simulink model "model"  (R2022b)
settings: Solver=VariableStepAuto  StartTime=0.0  StopTime=10  RelTol=1e-3
libraries: fuzblock x4, slpidlib x2
settings Model: Creator=Lenovo  LastModifiedBy=Lenovo

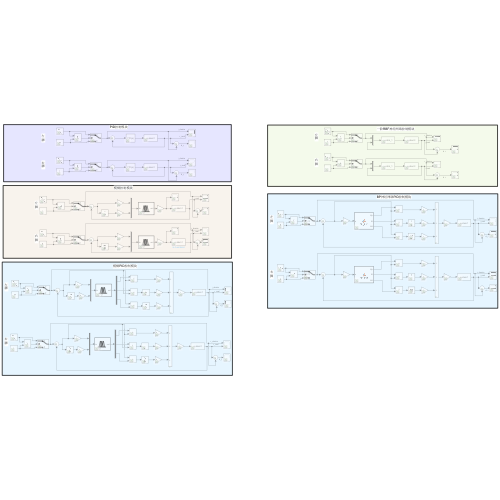
[thumbnail: Simulink's stored preview of the top-level diagram]
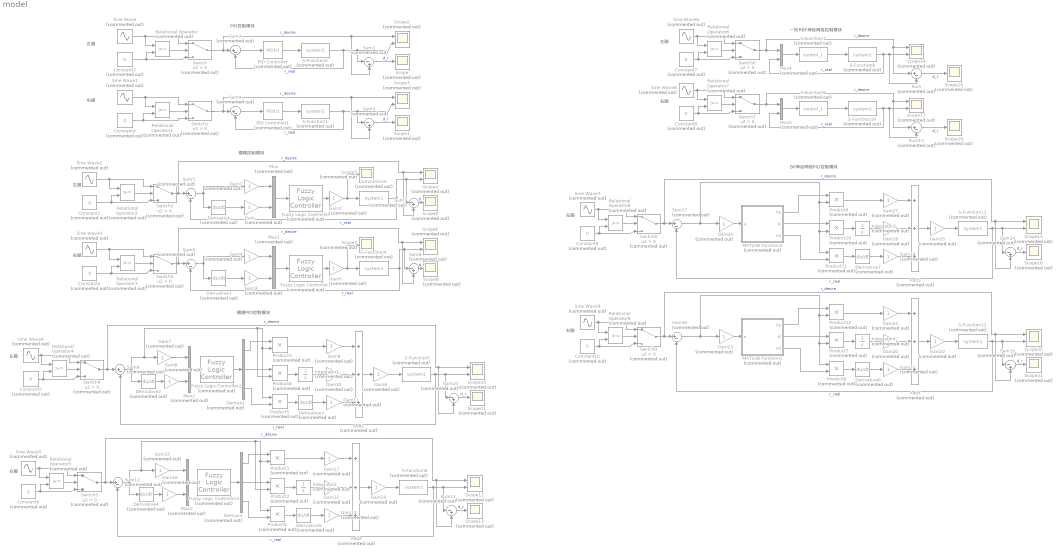
== system model ==
  note: 左脚
  note: PID控制模块
  note: 右脚
  note: 模糊控制模块
  note: 左脚
  note: 右脚
  note: 模糊PID控制模块
  note: 左脚
  note: 右脚
  note: 一阶RBF神经网络控制模块
  note: 左脚
  note: 右脚
  note: BP神经网络PID控制模块
  note: 左脚
  note: 右脚
  Add{1..4} (4 alike) : Sum  Commented=on  Inputs=+++
  Constant{1..10} (10 alike) : Constant  Commented=on  Value=0
  Demux1 : Demux  Commented=on  Outputs=3
  Demux2 : Demux  Commented=on  Outputs=3
  Derivative{,1..7} (8 alike) : Derivative  Commented=on
  Fuzzy Logic Controller : fuzblock/Fuzzy Logic  Controller  Commented=on  FIS='fuzzy1.fis'  OutputSampleNumber=101  DataType=double  FuzzifiedInputs=off  RuleFiringStrengths=off  RuleOutputs=off  AggregatedOutputs=off  SimulateUsing=Interpreted execution  OutOfRangeInputValueMessage=warning  NoRuleFiredMessage=warning  EmptyOutputFuzzySetMessage=warning
  Fuzzy Logic Controller1 : fuzblock/Fuzzy Logic  Controller  Commented=on  FIS='fuzzy1.fis'  OutputSampleNumber=101  DataType=double  FuzzifiedInputs=off  RuleFiringStrengths=off  RuleOutputs=off  AggregatedOutputs=off  SimulateUsing=Interpreted execution  OutOfRangeInputValueMessage=warning  NoRuleFiredMessage=warning  EmptyOutputFuzzySetMessage=warning
  Fuzzy Logic Controller2 : fuzblock/Fuzzy Logic  Controller  Commented=on  FIS='PIDfuzzy1.fis'  OutputSampleNumber=101  DataType=double  FuzzifiedInputs=off  RuleFiringStrengths=off  RuleOutputs=off  AggregatedOutputs=off  SimulateUsing=Interpreted execution  OutOfRangeInputValueMessage=warning  NoRuleFiredMessage=warning  EmptyOutputFuzzySetMessage=warning
  Fuzzy Logic Controller3 : fuzblock/Fuzzy Logic  Controller  Commented=on  FIS='PIDfuzzy1.fis'  OutputSampleNumber=101  DataType=double  FuzzifiedInputs=off  RuleFiringStrengths=off  RuleOutputs=off  AggregatedOutputs=off  SimulateUsing=Interpreted execution  OutOfRangeInputValueMessage=warning  NoRuleFiredMessage=warning  EmptyOutputFuzzySetMessage=warning
  Gain{,1..27} (28 alike) : Gain  Commented=on
  Integrator{1..4} (4 alike) : Integrator  Commented=on
  MATLAB Function1 : MATLAB Function  Commented=on  TreatAsAtomicUnit=on
  MATLAB Function2 : MATLAB Function  Commented=on  TreatAsAtomicUnit=on
  Mux{,1..5} (6 alike) : Mux  Commented=on  Inputs=2
  PID Controller : slpidlib/PID Controller  Commented=on  Controller=PID  Form=Parallel  TimeDomain=Continuous-time  UseExternalTs=off  SampleTime=-1  IntegratorMethod=Forward Euler  FilterMethod=Forward Euler  ControllerParametersSource=internal  P=871.012527892708  I=1996.38268425314  UseKiTs=off  D=84.4356751014045  N=44899.2539327158  UseFilter=on  TunerSelectOption=Transfer Function Based (PID Tuner App)  InitialConditionSource=internal  InitialConditionForIntegrator=0  InitialConditionForFilter=0  DifferentiatorICPrevScaledInput=0  ExternalReset=none  TrackingMode=off  Kt=1  LimitOutput=off  SatLimitsSource=internal  UpperSaturationLimit=inf  LowerSaturationLimit=-inf  LinearizeAsGain=on  AntiWindupMode=none  Kb=1  LimitIntegrator=off  UpperIntegratorSaturationLimit=inf  LowerIntegratorSaturationLimit=-inf  POutMin=[]  POutMax=[]  IOutMin=[]  IOutMax=[]  DOutMin=[]  DOutMax=[]  NOutMin=[]  NOutMax=[]  SumOutMin=[]  SumOutMax=[]  SaturationOutMin=[]  SaturationOutMax=[]  PParamMin=[]  PParamMax=[]  IParamMin=[]  IParamMax=[]  DParamMin=[]  DParamMax=[]  NParamMin=[]  NParamMax=[]  KbParamMin=[]  KbParamMax=[]  KtParamMin=[]  KtParamMax=[]  KbOutMin=[]  KbOutMax=[]  KtOutMin=[]  KtOutMax=[]  IntegratorOutMin=[]  IntegratorOutMax=[]  FilterOutMin=[]  FilterOutMax=[]  SumI1OutMin=[]  SumI1OutMax=[]  SumI2OutMin=[]  SumI2OutMax=[]  SumI3OutMin=[]  SumI3OutMax=[]  SumI4OutMin=[]  SumI4OutMax=[]  SumDOutMin=[]  SumDOutMax=[]  DifferentiatorOutMin=[]  DifferentiatorOutMax=[]  FilterDiffOutCoefMin=[]  FilterDiffOutCoefMax=[]  ReciprocalOutMin=[]  ReciprocalOutMax=[]  SumDenOutMin=[]  SumDenOutMax=[]  SumNumOutMin=[]  SumNumOutMax=[]  DivideOutMin=[]  DivideOutMax=[]  UdiffTsProdOutMin=[]  UdiffTsProdOutMax=[]  NTsProdOutMin=[]  NTsProdOutMax=[]  UintegralTsProdOutMin=[]  UintegralTsProdOutMax=[]  UngainTsProdOutMin=[]  UngainTsProdOutMax=[]  ClampingZeroOutDataTypeStr=Inherit: Inherit via back propagation  ClampingZeroOutMin=[]  ClampingZeroOutMax=[]  FilterDenConstantOutDataTypeStr=Inherit: Inherit via back propagation  FilterDenConstantOutMin=[]  FilterDenConstantOutMax=[]  PCopyOutDataTypeStr=Inherit: Inherit via back propagation  PCopyOutMin=[]  PCopyOutMax=[]  NCopyOutDataTypeStr=Inherit: Inherit via back propagation  NCopyOutMin=[]  NCopyOutMax=[]  IntegratorContinuousStateAttributes=''  IntegratorStateMustResolveToSignalObject=off  IntegratorRTWStateStorageClass=Auto  FilterContinuousStateAttributes=''  FilterStateMustResolveToSignalObject=off  FilterRTWStateStorageClass=Auto  ParallelPVariant=InternalParameters  IdealPVariant=Disabled  IVariant=InternalParameters  DVariant=InternalParameters  IntegratorVariant=Continuous  SatVariant=Disabled  AWVariant=Passthrough  PCopyVariant=Disabled  TRVariant=Disabled  FdbkBlocksVariant=Forward  IdealPFdbkVariant=Disabled  SatFdbkVariant=Disabled  DerivativeFilterVariant=ContFilter  NVariant=InternalParameters  NCopyVariant=Disabled  FilterICVariant=InternalICsFilter  IntegratorICVariant=InternalICs  ExternalResetVariant=Disabled  TRSumVariant=Passthrough  SumFdbkVariant=Disabled  SumVariant=Sum_PID  TsampFilterVariant=InternalTs  TsampNgainVariant=Passthrough  TsampIntegralVariant=Passthrough  ExternalSaturationOutDataTypeStr=Inherit: Same as second input
  PID Controller1 : slpidlib/PID Controller  Commented=on  Controller=PID  Form=Parallel  TimeDomain=Continuous-time  UseExternalTs=off  SampleTime=-1  IntegratorMethod=Forward Euler  FilterMethod=Forward Euler  ControllerParametersSource=internal  P=871.012527892708  I=1996.38268425314  UseKiTs=off  D=84.4356751014045  N=44899.2539327158  UseFilter=on  TunerSelectOption=Transfer Function Based (PID Tuner App)  InitialConditionSource=internal  InitialConditionForIntegrator=0  InitialConditionForFilter=0  DifferentiatorICPrevScaledInput=0  ExternalReset=none  TrackingMode=off  Kt=1  LimitOutput=off  SatLimitsSource=internal  UpperSaturationLimit=inf  LowerSaturationLimit=-inf  LinearizeAsGain=on  AntiWindupMode=none  Kb=1  LimitIntegrator=off  UpperIntegratorSaturationLimit=inf  LowerIntegratorSaturationLimit=-inf  POutMin=[]  POutMax=[]  IOutMin=[]  IOutMax=[]  DOutMin=[]  DOutMax=[]  NOutMin=[]  NOutMax=[]  SumOutMin=[]  SumOutMax=[]  SaturationOutMin=[]  SaturationOutMax=[]  PParamMin=[]  PParamMax=[]  IParamMin=[]  IParamMax=[]  DParamMin=[]  DParamMax=[]  NParamMin=[]  NParamMax=[]  KbParamMin=[]  KbParamMax=[]  KtParamMin=[]  KtParamMax=[]  KbOutMin=[]  KbOutMax=[]  KtOutMin=[]  KtOutMax=[]  IntegratorOutMin=[]  IntegratorOutMax=[]  FilterOutMin=[]  FilterOutMax=[]  SumI1OutMin=[]  SumI1OutMax=[]  SumI2OutMin=[]  SumI2OutMax=[]  SumI3OutMin=[]  SumI3OutMax=[]  SumI4OutMin=[]  SumI4OutMax=[]  SumDOutMin=[]  SumDOutMax=[]  DifferentiatorOutMin=[]  DifferentiatorOutMax=[]  FilterDiffOutCoefMin=[]  FilterDiffOutCoefMax=[]  ReciprocalOutMin=[]  ReciprocalOutMax=[]  SumDenOutMin=[]  SumDenOutMax=[]  SumNumOutMin=[]  SumNumOutMax=[]  DivideOutMin=[]  DivideOutMax=[]  UdiffTsProdOutMin=[]  UdiffTsProdOutMax=[]  NTsProdOutMin=[]  NTsProdOutMax=[]  UintegralTsProdOutMin=[]  UintegralTsProdOutMax=[]  UngainTsProdOutMin=[]  UngainTsProdOutMax=[]  ClampingZeroOutDataTypeStr=Inherit: Inherit via back propagation  ClampingZeroOutMin=[]  ClampingZeroOutMax=[]  FilterDenConstantOutDataTypeStr=Inherit: Inherit via back propagation  FilterDenConstantOutMin=[]  FilterDenConstantOutMax=[]  PCopyOutDataTypeStr=Inherit: Inherit via back propagation  PCopyOutMin=[]  PCopyOutMax=[]  NCopyOutDataTypeStr=Inherit: Inherit via back propagation  NCopyOutMin=[]  NCopyOutMax=[]  IntegratorContinuousStateAttributes=''  IntegratorStateMustResolveToSignalObject=off  IntegratorRTWStateStorageClass=Auto  FilterContinuousStateAttributes=''  FilterStateMustResolveToSignalObject=off  FilterRTWStateStorageClass=Auto  ParallelPVariant=InternalParameters  IdealPVariant=Disabled  IVariant=InternalParameters  DVariant=InternalParameters  IntegratorVariant=Continuous  SatVariant=Disabled  AWVariant=Passthrough  PCopyVariant=Disabled  TRVariant=Disabled  FdbkBlocksVariant=Forward  IdealPFdbkVariant=Disabled  SatFdbkVariant=Disabled  DerivativeFilterVariant=ContFilter  NVariant=InternalParameters  NCopyVariant=Disabled  FilterICVariant=InternalICsFilter  IntegratorICVariant=InternalICs  ExternalResetVariant=Disabled  TRSumVariant=Passthrough  SumFdbkVariant=Disabled  SumVariant=Sum_PID  TsampFilterVariant=InternalTs  TsampNgainVariant=Passthrough  TsampIntegralVariant=Passthrough  ExternalSaturationOutDataTypeStr=Inherit: Same as second input
  Product{1..12} (12 alike) : Product  Commented=on
  Relational Operator{,1..9} (10 alike) : RelationalOperator  Commented=on  OutDataTypeStr=boolean  RndMeth=Simplest  InputSameDT=off
  S-Function{1..6,8,10..12} (10 alike) : S-Function  Commented=on  FunctionName=system1  SFunctionDeploymentMode=off  EnableBusSupport=off
  S-Function7 : S-Function  Commented=on  FunctionName=control_1  SFunctionDeploymentMode=off  EnableBusSupport=off
  S-Function9 : S-Function  Commented=on  FunctionName=control_1  SFunctionDeploymentMode=off  EnableBusSupport=off
  Scope{,1,5,7..9,11,13,16,18..19,21} (12 alike) : Scope  Commented=on
  Scope{2..4,6,10,12,14..15,17,20} (10 alike) : Scope  Commented=on  NumInputPorts=2
  Sine Wave{,2,4,6..7} (5 alike) : Sin  Commented=on  SampleTime=0
  Sine Wave{1,3,5,8..9} (5 alike) : Sin  Commented=on  Phase=pi  SampleTime=0
  Sum{,2,4..6,9,12..13,16..17} (10 alike) : Sum  Commented=on  Inputs=|+-
  Sum{1,3,7..8,10..11,14..15} (8 alike) : Sum  Commented=on  Inputs=|-+
  Switch{,1..9} (10 alike) : Switch  Commented=on  Criteria=u2 > Threshold  SaturateOnIntegerOverflow=off  InputSameDT=off
  wires:
  S-Function2/1 -> Scope2/2, Sum1/1, Sum2/2  "r_real"
  Switch/1 -> Scope2/1, Sum1/2, Sum2/1  "r_desire"
  PID Controller/1 -> S-Function2/1
  Sum2/1 -> PID Controller/1
  Sum1/1 -> Scope/1  "d_r"
  Switch1/1 -> Scope3/1, Sum3/2, Sum4/1  "r_desire"
  PID Controller1/1 -> S-Function1/1
  Sum3/1 -> Scope1/1  "d_r"
  S-Function1/1 -> Sum3/1, Scope3/2, Sum4/2  "r_real"
  Sum4/1 -> PID Controller1/1
  Relational Operator/1 -> Switch/2
  Sine Wave/1 -> Switch/1, Relational Operator/1
  Constant3/1 -> Relational Operator/2, Switch/3
  Relational Operator1/1 -> Switch1/2
  Sine Wave1/1 -> Switch1/1, Relational Operator1/1
  Constant4/1 -> Switch1/3, Relational Operator1/2
  Gain2/1 -> Scope5/1, S-Function3/1
  Derivative/1 -> Gain/1
  Gain/1 -> Mux/2
  Gain1/1 -> Mux/1
  S-Function3/1 -> Scope4/2, Sum7/1, Sum5/2  "r_real"
  Mux/1 -> Fuzzy Logic Controller/1
  Switch2/1 -> Sum7/2, Scope4/1, Sum5/1  "r_desire"
  Sum5/1 -> Derivative/1, Gain1/1
  Fuzzy Logic Controller/1 -> Gain2/1
  Sine Wave2/1 -> Switch2/1, Relational Operator2/1
  Relational Operator2/1 -> Switch2/2
  Constant1/1 -> Relational Operator2/2, Switch2/3
  Switch3/1 -> Scope6/1, Sum8/2, Sum6/1  "r_desire"
  Constant2/1 -> Relational Operator3/2, Switch3/3
  Relational Operator3/1 -> Switch3/2
  Sum6/1 -> Derivative1/1, Gain4/1
  Fuzzy Logic Controller1/1 -> Gain5/1
  Mux1/1 -> Fuzzy Logic Controller1/1
  Gain5/1 -> Scope7/1, S-Function4/1
  Gain3/1 -> Mux1/2
  Sine Wave3/1 -> Switch3/1, Relational Operator3/1
  Gain4/1 -> Mux1/1
  S-Function4/1 -> Sum6/2, Sum8/1, Scope6/2  "r_real"
  Derivative1/1 -> Gain3/1
  Sum7/1 -> Scope9/1  "d_r"
  Sum8/1 -> Scope8/1  "d_r"
  Derivative3/1 -> Gain11/1
  Gain8/1 -> Mux2/2
  Product4/1 -> Integrator1/1
  Product3/1 -> Gain9/1
  Add1/1 -> Gain6/1
  Sum9/1 -> Derivative2/1, Product5/1, Product3/2, Product4/2, Gain7/1
  Demux2/2 -> Product4/1
  Demux2/3 -> Product5/2
  Derivative2/1 -> Gain8/1
  Demux2/1 -> Product3/1
  Integrator1/1 -> Gain10/1
  Product5/1 -> Derivative3/1
  Gain7/1 -> Mux2/1
  Gain6/1 -> S-Function5/1
  Fuzzy Logic Controller2/1 -> Demux2/1
  S-Function5/1 -> Sum9/2, Sum10/1, Scope10/2  "r_real"
  Gain11/1 -> Add1/3
  Mux2/1 -> Fuzzy Logic Controller2/1
  Gain10/1 -> Add1/2
  Gain9/1 -> Add1/1
  Sine Wave4/1 -> Switch4/1, Relational Operator4/1
  Relational Operator4/1 -> Switch4/2
  Constant5/1 -> Relational Operator4/2, Switch4/3
  Sum10/1 -> Scope11/1  "d_r"
  Switch4/1 -> Sum10/2, Scope10/1, Sum9/1  "r_desire"
  Constant6/1 -> Relational Operator5/2, Switch5/3
  Sine Wave5/1 -> Switch5/1, Relational Operator5/1
  Relational Operator5/1 -> Switch5/2
  Sum11/1 -> Scope13/1  "d_r"
  Gain14/1 -> S-Function6/1
  Switch5/1 -> Sum11/2, Scope12/1, Sum12/1  "r_desire"
  Mux3/1 -> Fuzzy Logic Controller3/1
  Gain13/1 -> Add2/3
  Fuzzy Logic Controller3/1 -> Demux1/1
  S-Function6/1 -> Sum12/2, Sum11/1, Scope12/2  "r_real"
  Demux1/1 -> Product1/1
  Derivative4/1 -> Gain16/1
  Gain12/1 -> Add2/2
  Demux1/2 -> Product2/1
  Demux1/3 -> Product6/2
  Integrator2/1 -> Gain12/1
  Product6/1 -> Derivative5/1
  Sum12/1 -> Derivative4/1, Product6/1, Product1/2, Product2/2, Gain15/1
  Gain17/1 -> Add2/1
  Gain15/1 -> Mux3/1
  Gain16/1 -> Mux3/2
  Product1/1 -> Gain17/1
  Product2/1 -> Integrator2/1
  Add2/1 -> Gain14/1
  Derivative5/1 -> Gain13/1
  Sum/1 -> Scope16/1  "d_r"
  Mux4/1 -> S-Function7/1
  S-Function7/1 -> S-Function8/1
  S-Function8/1 -> Mux4/2, Scope14/2, Sum/2  "r_real"
  Switch6/1 -> Scope14/1, Sum/1, Mux4/1  "r_desire"
  Constant7/1 -> Relational Operator6/2, Switch6/3
  Relational Operator6/1 -> Switch6/2
  Sine Wave6/1 -> Switch6/1, Relational Operator6/1
  Switch7/1 -> Scope17/1, Sum13/1, Mux5/1  "r_desire"
  Constant8/1 -> Relational Operator7/2, Switch7/3
  Sine Wave8/1 -> Switch7/1, Relational Operator7/1
  Relational Operator7/1 -> Switch7/2
  S-Function10/1 -> Mux5/2, Scope17/2, Sum13/2  "r_real"
  S-Function9/1 -> S-Function10/1
  Sum13/1 -> Scope19/1  "d_r"
  Mux5/1 -> S-Function9/1
  MATLAB Function1/3(Kd) -> Product8/2
  MATLAB Function1/1(Kp) -> Product12/1
  Sum16/1 -> Product7/2, Product8/1, Product12/2, Gain23/1
  Gain20/1 -> Add4/2
  Gain22/1 -> S-Function12/1
  Sine Wave9/1 -> Switch9/1, Relational Operator9/1
  Product12/1 -> Gain24/1
  Product8/1 -> Derivative6/1
  Gain21/1 -> Add4/3
  Add4/1 -> Gain22/1
  Product7/1 -> Integrator4/1
  Integrator4/1 -> Gain20/1
  Relational Operator9/1 -> Switch9/2
  Constant10/1 -> Relational Operator9/2, Switch9/3
  Sum15/1 -> Scope21/1  "d_r"
  Switch9/1 -> Sum15/2, Scope20/1, Sum16/1  "r_desire"
  S-Function12/1 -> Sum16/2, Sum15/1, Scope20/2  "r_real"
  MATLAB Function1/2(Ki) -> Product7/1
  Gain23/1 -> MATLAB Function1/1(e)
  Gain24/1 -> Add4/1
  Derivative6/1 -> Gain21/1
  Relational Operator8/1 -> Switch8/2
  Gain26/1 -> MATLAB Function2/1(e)
  Gain18/1 -> Add3/2
  Sine Wave7/1 -> Switch8/1, Relational Operator8/1
  Switch8/1 -> Sum14/2, Scope15/1, Sum17/1  "r_desire"
  Gain19/1 -> Add3/3
  MATLAB Function2/2(Ki) -> Product10/1
  Constant9/1 -> Relational Operator8/2, Switch8/3
  Product9/1 -> Gain27/1
  Gain27/1 -> Add3/1
  Gain25/1 -> S-Function11/1
  Derivative7/1 -> Gain19/1
  Product11/1 -> Derivative7/1
  Sum14/1 -> Scope18/1  "d_r"
  MATLAB Function2/1(Kp) -> Product9/1
  Integrator3/1 -> Gain18/1
  Product10/1 -> Integrator3/1
  S-Function11/1 -> Sum17/2, Sum14/1, Scope15/2  "r_real"
  Sum17/1 -> Product10/2, Product11/1, Product9/2, Gain26/1
  Add3/1 -> Gain25/1
  MATLAB Function2/3(Kd) -> Product11/2

== matlab function model/MATLAB Function2 ==
  settings: updateMethod=DISCRETE
  data: e input; Kp output; Ki output; Kd output
function [Kp, Ki, Kd] = BP_PID(e)
% BPNeuralPID - 使用 BP 神经网络在线调整 PID 参数的示例
%
% 输入:
%   e  : 当前位置误差
%
% 输出:
%   Kp : PID 比例增益
%   Ki : PID 积分增益
%   Kd : PID 微分增益
%
% 说明:
%   该函数使用一个两层的前馈 BP 神经网络 (1 个隐藏层)。
%   前向传播: e -> (隐藏层) -> [Kp, Ki, Kd]
%   反向传播: 根据训练误差调整网络权重和偏置。

    %-------------------------------------------------------
    % 1. 定义输入向量
    %-------------------------------------------------------
    inVec = e;  % 单一输入: 误差 e
    
    %-------------------------------------------------------
    % 2. 声明并初始化(若为空)网络参数: W1, b1, W2, b2
    %   使用 persistent 来保存状态，以便在每次函数调用之间“记住”网络参数
    %-------------------------------------------------------
    persistent W1 b1 W2 b2 learning_rate
    
    if isempty(W1)
        %---------------网络结构超参数可自行修改---------------
        input_size   = 1;    % 输入层神经元个数 (仅 e)
        hidden_size  = 5000;   % 隐藏层神经元个数
        output_size  = 3;    % 输出层神经元个数 (Kp, Ki, Kd)
        
        % 初始化权重和偏置 (建议较小的随机值以避免激活函数饱和)
        W1 = rand(input_size, hidden_size) * 0.1; 
        b1 = rand(1, hidden_size) * 0.1;
        W2 = rand(hidden_size, output_size) * 0.1;
        b2 = rand(1, output_size) * 0.1;
        
        learning_rate = 0.01; % 学习率，可根据实际需求调整
    end
    
    %-------------------------------------------------------
    % 3. 前向传播 (Forward Pass)
    %-------------------------------------------------------
    % 隐藏层线性变换
    z1 = inVec * W1 + b1;   
    % 隐藏层激活 (Sigmoid 或其他激活函数)
    a1 = sigmoid(z1);
    
    % 输出层线性变换 (可选择性添加激活函数)
    z2 = a1 * W2 + b2;
    a2 = z2;  % 直接使用线性输出
    
    % 从网络输出中获取 PID 参数
    Kp = a2(1);
    Ki = a2(2);
    Kd = a2(3);
    
    %-------------------------------------------------------
    % 4. 计算训练误差并反向传播 (Backward Pass)
    %-------------------------------------------------------
    % 计算输出层误差
    err_output = a2 - [Kp,Ki,Kd];   % 尺寸: 1 x 3
    
    % 输出层对 z2 的偏导(线性激活，导数为1)
    dZ2 = err_output; 
    % 输出层权重梯度和偏置梯度
    dW2 = a1' * dZ2;            % (hidden_size x 1) * (1 x output_size) = (hidden_size x output_size)
    db2 = dZ2;                  % (1 x output_size)
    
    % 反向传播到隐藏层
    dA1 = dZ2 * W2';            % (1 x output_size) * (output_size x hidden_size) = (1 x hidden_size)
    % 隐藏层 sigmoid 激活的梯度
    dZ1 = dA1 .* sigmoid_derivative(a1);  % element-wise
    % 隐藏层到输入层权重梯度和偏置梯度
    dW1 = inVec' * dZ1;         % (1 x 1) * (1 x hidden_size) = (1 x hidden_size)
    db1 = dZ1;                  % (1 x hidden_size)
    
    %-------------------------------------------------------
    % 5. 更新网络权重和偏置
    %-------------------------------------------------------
    W2 = W2 - learning_rate * dW2;
    b2 = b2 - learning_rate * db2;
    W1 = W1 - learning_rate * dW1;
    b1 = b1 - learning_rate * db1;
    
    %-------------------------------------------------------
    % 辅助函数: Sigmoid 及其导数
    %-------------------------------------------------------
    function y = sigmoid(x)
        y = 1 ./ (1 + exp(-x));
    end

    function y = sigmoid_derivative(x)
        y = x .* (1 - x);
    end

end

== matlab function model/MATLAB Function1 ==
  settings: updateMethod=DISCRETE
  data: e input; Kp output; Ki output; Kd output
function [Kp, Ki, Kd] = BP_PID(e)
% BPNeuralPID - 使用 BP 神经网络在线调整 PID 参数的示例
%
% 输入:
%   e  : 当前位置误差
%
% 输出:
%   Kp : PID 比例增益
%   Ki : PID 积分增益
%   Kd : PID 微分增益
%
% 说明:
%   该函数使用一个两层的前馈 BP 神经网络 (1 个隐藏层)。
%   前向传播: e -> (隐藏层) -> [Kp, Ki, Kd]
%   反向传播: 根据训练误差调整网络权重和偏置。

    %-------------------------------------------------------
    % 1. 定义输入向量
    %-------------------------------------------------------
    inVec = e;  % 单一输入: 误差 e
    
    %-------------------------------------------------------
    % 2. 声明并初始化(若为空)网络参数: W1, b1, W2, b2
    %   使用 persistent 来保存状态，以便在每次函数调用之间“记住”网络参数
    %-------------------------------------------------------
    persistent W1 b1 W2 b2 learning_rate
    
    if isempty(W1)
        %---------------网络结构超参数可自行修改---------------
        input_size   = 1;    % 输入层神经元个数 (仅 e)
        hidden_size  = 5000;   % 隐藏层神经元个数
        output_size  = 3;    % 输出层神经元个数 (Kp, Ki, Kd)
        
        % 初始化权重和偏置 (建议较小的随机值以避免激活函数饱和)
        W1 = rand(input_size, hidden_size) * 0.1; 
        b1 = rand(1, hidden_size) * 0.1;
        W2 = rand(hidden_size, output_size) * 0.1;
        b2 = rand(1, output_size) * 0.1;
        
        learning_rate = 0.01; % 学习率，可根据实际需求调整
    end
    
    %-------------------------------------------------------
    % 3. 前向传播 (Forward Pass)
    %-------------------------------------------------------
    % 隐藏层线性变换
    z1 = inVec * W1 + b1;   
    % 隐藏层激活 (Sigmoid 或其他激活函数)
    a1 = sigmoid(z1);
    
    % 输出层线性变换 (可选择性添加激活函数)
    z2 = a1 * W2 + b2;
    a2 = z2;  % 直接使用线性输出
    
    % 从网络输出中获取 PID 参数
    Kp = a2(1);
    Ki = a2(2);
    Kd = a2(3);
    
    %-------------------------------------------------------
    % 4. 计算训练误差并反向传播 (Backward Pass)
    %-------------------------------------------------------
    % 计算输出层误差
    err_output = a2 - [Kp,Ki,Kd];   % 尺寸: 1 x 3
    
    % 输出层对 z2 的偏导(线性激活，导数为1)
    dZ2 = err_output; 
    % 输出层权重梯度和偏置梯度
    dW2 = a1' * dZ2;            % (hidden_size x 1) * (1 x output_size) = (hidden_size x output_size)
    db2 = dZ2;                  % (1 x output_size)
    
    % 反向传播到隐藏层
    dA1 = dZ2 * W2';            % (1 x output_size) * (output_size x hidden_size) = (1 x hidden_size)
    % 隐藏层 sigmoid 激活的梯度
    dZ1 = dA1 .* sigmoid_derivative(a1);  % element-wise
    % 隐藏层到输入层权重梯度和偏置梯度
    dW1 = inVec' * dZ1;         % (1 x 1) * (1 x hidden_size) = (1 x hidden_size)
    db1 = dZ1;                  % (1 x hidden_size)
    
    %-------------------------------------------------------
    % 5. 更新网络权重和偏置
    %-------------------------------------------------------
    W2 = W2 - learning_rate * dW2;
    b2 = b2 - learning_rate * db2;
    W1 = W1 - learning_rate * dW1;
    b1 = b1 - learning_rate * db1;
    
    %-------------------------------------------------------
    % 辅助函数: Sigmoid 及其导数
    %-------------------------------------------------------
    function y = sigmoid(x)
        y = 1 ./ (1 + exp(-x));
    end

    function y = sigmoid_derivative(x)
        y = x .* (1 - x);
    end

end
